simulink model "six_phase_plant"  (R2024b)
settings: Solver=FixedStepAuto  StartTime=0  StopTime=Tend  FixedStep=Tsim  RelTol=1e-3
values from neighbouring files (symbols this model uses):
  alpha_s = 2*pi/m*ps    (= 5.23598775598)    [setup.m]
  alpha_t = 2*pi/m*p    (= 4.18879020479)    [setup.m]
  Cm = 2/m    (= 0.333333333333)    [setup.m]
  fx_cmd = 9    [setup.m]
  fx_end = 0.025    [setup.m]
  fx_start = 0.002    [setup.m]
  fy_cmd = -4.5    [setup.m]
  fy_end = 0.025    [setup.m]
  fy_start = 0.001    [setup.m]
  id_cmd = 0    [setup.m]
  id_end = 0.025    [setup.m]
  id_start = 0    [setup.m]
  Ke = 0.003    [setup.m]
  Kf = 1.8    [setup.m]
  Ki_s = R*wb    (= 942.477796077)    [setup.m]
  Ki_t = R*wb    (= 942.477796077)    [setup.m]
  Kp_s = Ls*wb    (= 1.41371669412)    [setup.m]
  Kp_t = Lt*wb    (= 0.942477796077)    [setup.m]
  Kt = 0.02    [setup.m]
  Ls = L_alpha_beta(3,3)    [setup.m]
  Lt = L_alpha_beta(1,1)    [setup.m]
  p = 4    [setup.m]
  speed_cmd = 7500    [setup.m]
  torque_cmd = 0.2    [setup.m]
  torque_end = 0.025    [setup.m]
  torque_start = 0.002    [setup.m]
settings Model: Creator=chiba  LastModifiedBy=tnoguchi
settings SolverCC: AllowMultiTaskInputOutput=on
settings OptimizationCC: DefaultParameterBehavior=Inlined  ReuseModelBlockBuffer=off  EnhancedBackFolding=on  PassReuseOutputArgsAs=Individual arguments  ZeroExternalMemoryAtStartup=off  ZeroInternalMemoryAtStartup=off  OptimizeBlockOrder=speed  DifferentSizesBufferReuse=on  EfficientTunableParamExpr=on
settings DebuggingCC: ParameterTunabilityLossMsg=error
settings SFSimCC: MATLABDynamicMemAlloc=off
settings RTWCC: Description=Embedded Coder  SystemTargetFile=ert.tlc  TemplateMakefile=ert_default_tmf  GPUComputeCapability=3.5
settings CodeAppCC: ForceParamTrailComments=on  IgnoreCustomStorageClasses=off  OperatorAnnotations=on  SimulinkDataObjDesc=on  SFDataObjDesc=on  InsertBlockDesc=on
settings ERTTargetCC: TargetLangStandard=C99 (ISO)  ERTCustomFileTemplate=example_file_process.tlc  DynamicArrayContainerType=coder::array

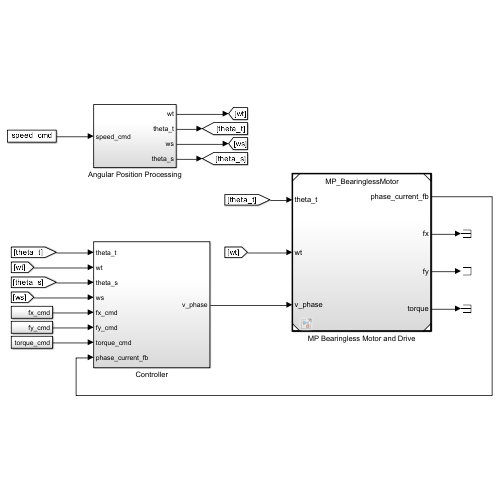
[thumbnail: Simulink's stored preview of the top-level diagram]
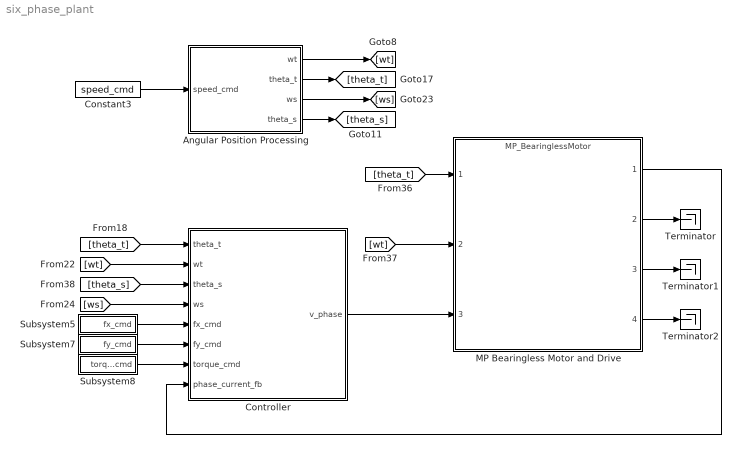
== system six_phase_plant ==
  Angular Position Processing : Subsystem
  Constant3 : Constant  Value=speed_cmd
  Controller : Subsystem
  MP Bearingless Motor and Drive : ModelReference  ModelNameDialog=MP_BearinglessMotor  SimulationMode=Normal  ModelReferenceVersion=5.215
  Subsystem5 : Subsystem
  Subsystem7 : Subsystem
  Subsystem8 : Subsystem
  Terminator : Terminator
  Terminator1 : Terminator
  Terminator2 : Terminator
  wires:
  Constant3/1 -> Angular Position Processing/1(speed_cmd)
  Angular Position Processing/1(wt) -> [wt]
  Angular Position Processing/2(theta_t) -> [theta_t]
  Angular Position Processing/3(ws) -> [ws]
  Angular Position Processing/4(theta_s) -> [theta_s]
  [wt] -> MP Bearingless Motor and Drive/2
  [theta_t] -> MP Bearingless Motor and Drive/1
  [theta_t] -> Controller/1(theta_t)
  [wt] -> Controller/2(wt)
  [theta_s] -> Controller/3(theta_s)
  [ws] -> Controller/4(ws)
  Subsystem5/1(fx_cmd) -> Controller/5(fx_cmd)
  Subsystem7/1(fy_cmd) -> Controller/6(fy_cmd)
  Subsystem8/1(torque_cmd) -> Controller/7(torque_cmd)
  Controller/1(v_phase) -> MP Bearingless Motor and Drive/3
  MP Bearingless Motor and Drive/2 -> Terminator/1
  MP Bearingless Motor and Drive/3 -> Terminator1/1
  MP Bearingless Motor and Drive/4 -> Terminator2/1
  MP Bearingless Motor and Drive/1 -> Controller/8(phase_current_fb)

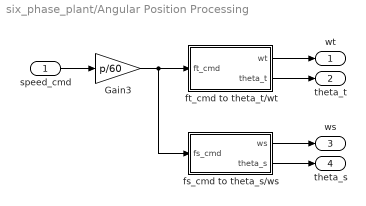
== system six_phase_plant/Angular Position Processing ==
  speed_cmd : Inport
  Gain3 : Gain  Gain=p/60
  fs_cmd to theta_s/ws : Subsystem
  ft_cmd to theta_t/wt : Subsystem
  wt : Outport
  theta_t : Outport  Port=2
  ws : Outport  Port=3
  theta_s : Outport  Port=4
  wires:
  ft_cmd to theta_t/wt/1(wt) -> wt/1
  fs_cmd to theta_s/ws/1(ws) -> ws/1
  Gain3/1 -> fs_cmd to theta_s/ws/1(fs_cmd), ft_cmd to theta_t/wt/1(ft_cmd)
  speed_cmd/1 -> Gain3/1
  ft_cmd to theta_t/wt/2(theta_t) -> theta_t/1
  fs_cmd to theta_s/ws/2(theta_s) -> theta_s/1

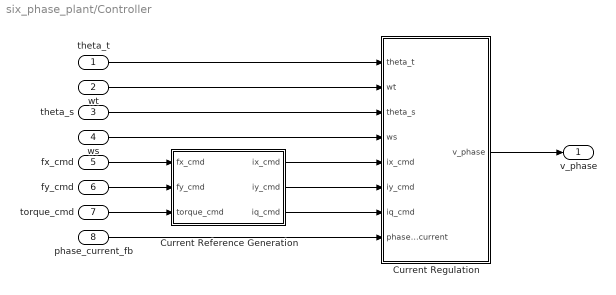
== system six_phase_plant/Controller ==
  theta_t : Inport
  wt : Inport  Port=2
  theta_s : Inport  Port=3
  ws : Inport  Port=4
  fx_cmd : Inport  Port=5
  fy_cmd : Inport  Port=6
  torque_cmd : Inport  Port=7
  phase_current_fb : Inport  Port=8
  Current Reference Generation : Subsystem
  Current Regulation : Subsystem
  v_phase : Outport
  wires:
  Current Reference Generation/3(iq_cmd) -> Current Regulation/7(iq_cmd)
  fy_cmd/1 -> Current Reference Generation/2(fy_cmd)
  torque_cmd/1 -> Current Reference Generation/3(torque_cmd)
  fx_cmd/1 -> Current Reference Generation/1(fx_cmd)
  Current Reference Generation/2(iy_cmd) -> Current Regulation/6(iy_cmd)
  theta_t/1 -> Current Regulation/1(theta_t)
  phase_current_fb/1 -> Current Regulation/8(phase_current)
  Current Regulation/1(v_phase) -> v_phase/1
  Current Reference Generation/1(ix_cmd) -> Current Regulation/5(ix_cmd)
  theta_s/1 -> Current Regulation/3(theta_s)
  ws/1 -> Current Regulation/4(ws)
  wt/1 -> Current Regulation/2(wt)

== system six_phase_plant/Subsystem5 ==
  Sum2 : Sum  Inputs=|++
  step : Step  Time=fx_start  After=fx_cmd  SampleTime=0
  step1 : Step  Time=fx_end  After=-fx_cmd  SampleTime=0
  fx_cmd : Outport
  wires:
  step1/1 -> Sum2/2
  step/1 -> Sum2/1
  Sum2/1 -> fx_cmd/1

== system six_phase_plant/Subsystem7 ==
  Sum2 : Sum  Inputs=|++
  step : Step  Time=fy_start  After=fy_cmd  SampleTime=0
  step1 : Step  Time=fy_end  After=-fy_cmd  SampleTime=0
  fy_cmd : Outport
  wires:
  step1/1 -> Sum2/2
  step/1 -> Sum2/1
  Sum2/1 -> fy_cmd/1

== system six_phase_plant/Subsystem8 ==
  Sum2 : Sum  Inputs=|++
  step : Step  Time=torque_start  After=torque_cmd  SampleTime=0
  step1 : Step  Time=torque_end  After=-torque_cmd  SampleTime=0
  torque_cmd : Outport
  wires:
  step1/1 -> Sum2/2
  step/1 -> Sum2/1
  Sum2/1 -> torque_cmd/1

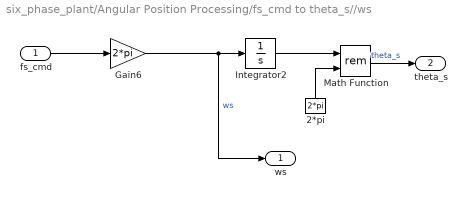
== system six_phase_plant/Angular Position Processing/fs_cmd to theta_s//ws ==
  fs_cmd : Inport
  2*pi : Constant  Value=2*pi
  Gain6 : Gain  Gain=2*pi
  Integrator2 : Integrator
  Math Function : Math  Operator=rem  SignedPower=on
  ws : Outport
  theta_s : Outport  Port=2
  wires:
  Gain6/1 -> ws/1, Integrator2/1  "ws"
  2*pi/1 -> Math Function/2
  fs_cmd/1 -> Gain6/1
  Integrator2/1 -> Math Function/1
  Math Function/1 -> theta_s/1  "theta_s"

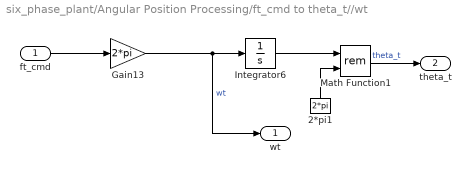
== system six_phase_plant/Angular Position Processing/ft_cmd to theta_t//wt ==
  ft_cmd : Inport
  2*pi1 : Constant  Value=2*pi
  Gain13 : Gain  Gain=2*pi
  Integrator6 : Integrator
  Math Function1 : Math  Operator=rem  SignedPower=on
  wt : Outport
  theta_t : Outport  Port=2
  wires:
  Integrator6/1 -> Math Function1/1
  ft_cmd/1 -> Gain13/1
  2*pi1/1 -> Math Function1/2
  Gain13/1 -> wt/1, Integrator6/1  "wt"
  Math Function1/1 -> theta_t/1  "theta_t"

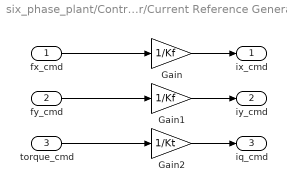
== system six_phase_plant/Controller/Current Reference Generation ==
  fx_cmd : Inport
  fy_cmd : Inport  Port=2
  torque_cmd : Inport  Port=3
  Gain : Gain  Gain=1/Kf
  Gain1 : Gain  Gain=1/Kf
  Gain2 : Gain  Gain=1/Kt
  ix_cmd : Outport
  iy_cmd : Outport  Port=2
  iq_cmd : Outport  Port=3
  wires:
  fx_cmd/1 -> Gain/1
  Gain2/1 -> iq_cmd/1
  Gain1/1 -> iy_cmd/1
  fy_cmd/1 -> Gain1/1
  torque_cmd/1 -> Gain2/1
  Gain/1 -> ix_cmd/1

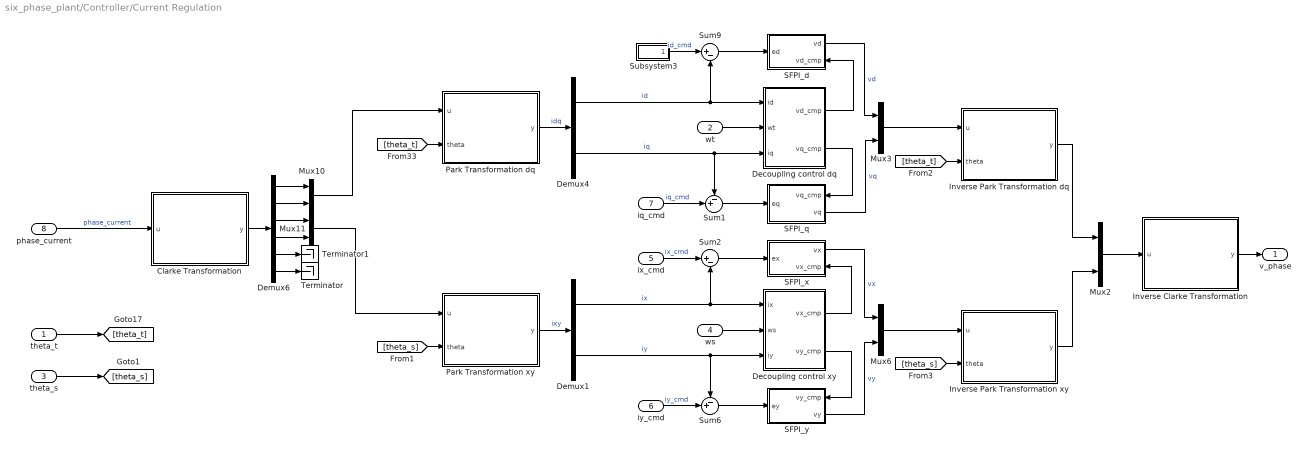
== system six_phase_plant/Controller/Current Regulation ==
  theta_t : Inport
  wt : Inport  Port=2
  theta_s : Inport  Port=3
  ws : Inport  Port=4
  ix_cmd : Inport  Port=5
  iy_cmd : Inport  Port=6
  iq_cmd : Inport  Port=7
  phase_current : Inport  Port=8
  Clarke Transformation : MATLAB Function  TreatAsAtomicUnit=on
  Decoupling control dq : Subsystem
  Decoupling control xy : Subsystem
  Demux1 : Demux  Outputs=2
  Demux4 : Demux  Outputs=2
  Demux6 : Demux  Outputs=6
  Inverse Clarke Transformation : MATLAB Function  TreatAsAtomicUnit=on
  Inverse Park Transformation dq : MATLAB Function  TreatAsAtomicUnit=on
  Inverse Park Transformation xy : MATLAB Function  TreatAsAtomicUnit=on
  Mux{2..3,6,10..11} (5 alike) : Mux  Inputs=2
  Park Transformation dq : MATLAB Function  TreatAsAtomicUnit=on
  Park Transformation xy : MATLAB Function  TreatAsAtomicUnit=on
  SFPI_d : Subsystem
      settings: PortSchema="{\"entries\":[{\"content\":{\"sides\":[{\"content\":{\"connectorIds\":[\"In1\"]},\"type\":\"ConnectorPlacement.EquallySpacedRectSide\",\"uuid\":\"0c9b1a56-be5b-4008-a4be-2c96991c93df\"},{\"content\":{\"connectorIds\":[\"Out1\",\"In2\"],\"side\":\"RIGHT\"},\"type\":\"ConnectorPlacement.EquallySpacedRectSide\",\"uuid\":\"62f10227-e6d2-436b-83cf-88635ef632ae\"},{\"content\":{\"side\":\"TOP\"},\"type\":\"ConnectorPlacement.EquallySpacedRectSide\",\"uuid\":\"775f088e-b169-44e0-8f62-950b5ccb7049\"}]},\"type\":\"ConnectorPlacement.EquallySpacedConnector\",\"uuid\":\"a91bb4f4-db64-42d6-b57d-9e899cd3ff7e\"}],\"packageUris\":[\"http://schema.mathworks.com/mf0/Connector/R2020b\"],\"version\":\"1.0\"}"
  SFPI_q : Subsystem
      settings: PortSchema="{\"entries\":[{\"content\":{\"sides\":[{\"content\":{\"connectorIds\":[\"In1\"]},\"type\":\"ConnectorPlacement.EquallySpacedRectSide\",\"uuid\":\"0c9b1a56-be5b-4008-a4be-2c96991c93df\"},{\"content\":{\"connectorIds\":[\"In2\",\"Out1\"],\"side\":\"RIGHT\"},\"type\":\"ConnectorPlacement.EquallySpacedRectSide\",\"uuid\":\"62f10227-e6d2-436b-83cf-88635ef632ae\"},{\"content\":{\"side\":\"TOP\"},\"type\":\"ConnectorPlacement.EquallySpacedRectSide\",\"uuid\":\"775f088e-b169-44e0-8f62-950b5ccb7049\"}]},\"type\":\"ConnectorPlacement.EquallySpacedConnector\",\"uuid\":\"a91bb4f4-db64-42d6-b57d-9e899cd3ff7e\"}],\"packageUris\":[\"http://schema.mathworks.com/mf0/Connector/R2020b\"],\"version\":\"1.0\"}"
  SFPI_x : Subsystem
      settings: PortSchema="{\"entries\":[{\"content\":{\"sides\":[{\"content\":{\"connectorIds\":[\"In1\"]},\"type\":\"ConnectorPlacement.EquallySpacedRectSide\",\"uuid\":\"0c9b1a56-be5b-4008-a4be-2c96991c93df\"},{\"content\":{\"connectorIds\":[\"Out1\",\"In2\"],\"side\":\"RIGHT\"},\"type\":\"ConnectorPlacement.EquallySpacedRectSide\",\"uuid\":\"62f10227-e6d2-436b-83cf-88635ef632ae\"},{\"content\":{\"side\":\"TOP\"},\"type\":\"ConnectorPlacement.EquallySpacedRectSide\",\"uuid\":\"775f088e-b169-44e0-8f62-950b5ccb7049\"}]},\"type\":\"ConnectorPlacement.EquallySpacedConnector\",\"uuid\":\"a91bb4f4-db64-42d6-b57d-9e899cd3ff7e\"}],\"packageUris\":[\"http://schema.mathworks.com/mf0/Connector/R2020b\"],\"version\":\"1.0\"}"
  SFPI_y : Subsystem
      settings: PortSchema="{\"entries\":[{\"content\":{\"sides\":[{\"content\":{\"connectorIds\":[\"In1\"]},\"type\":\"ConnectorPlacement.EquallySpacedRectSide\",\"uuid\":\"0c9b1a56-be5b-4008-a4be-2c96991c93df\"},{\"content\":{\"connectorIds\":[\"In2\",\"Out1\"],\"side\":\"RIGHT\"},\"type\":\"ConnectorPlacement.EquallySpacedRectSide\",\"uuid\":\"62f10227-e6d2-436b-83cf-88635ef632ae\"},{\"content\":{\"side\":\"TOP\"},\"type\":\"ConnectorPlacement.EquallySpacedRectSide\",\"uuid\":\"775f088e-b169-44e0-8f62-950b5ccb7049\"}]},\"type\":\"ConnectorPlacement.EquallySpacedConnector\",\"uuid\":\"a91bb4f4-db64-42d6-b57d-9e899cd3ff7e\"}],\"packageUris\":[\"http://schema.mathworks.com/mf0/Connector/R2020b\"],\"version\":\"1.0\"}"
  Subsystem3 : Subsystem
  Sum1 : Sum  Inputs=-+|
  Sum2 : Sum  Inputs=|+-
  Sum6 : Sum  Inputs=-+|
  Sum9 : Sum  Inputs=|+-
  Terminator : Terminator
  Terminator1 : Terminator
  v_phase : Outport
  wires:
  Park Transformation dq/1(y) -> Demux4/1  "idq"
  Demux6/1 -> Mux10/1
  Decoupling control dq/1(vd_cmp) -> SFPI_d/2(vd_cmp)
  ws/1 -> Decoupling control xy/2(ws)
  SFPI_y/1(vy) -> Mux6/2  "vy"
  Decoupling control dq/2(vq_cmp) -> SFPI_q/2(vq_cmp)
  Decoupling control xy/1(vx_cmp) -> SFPI_x/2(vx_cmp)
  Demux1/2 -> Sum6/1, Decoupling control xy/3(iy)  "iy"
  Mux2/1 -> Inverse Clarke Transformation/1(u)
  Mux3/1 -> Inverse Park Transformation dq/1(u)
  Mux11/1 -> Park Transformation xy/1(u)
  Mux6/1 -> Inverse Park Transformation xy/1(u)
  Demux6/3 -> Mux11/1
  Sum6/1 -> SFPI_y/1(ey)
  Demux6/4 -> Mux11/2
  Demux4/1 -> Sum9/2, Decoupling control dq/1(id)  "id"
  Decoupling control xy/2(vy_cmp) -> SFPI_y/2(vy_cmp)
  phase_current/1 -> Clarke Transformation/1(u)  "phase_current"
  Demux1/1 -> Sum2/2, Decoupling control xy/1(ix)  "ix"
  SFPI_x/1(vx) -> Mux6/1  "vx"
  SFPI_q/1(vq) -> Mux3/2  "vq"
  ix_cmd/1 -> Sum2/1  "ix_cmd"
  Demux6/5 -> Terminator1/1
  Demux4/2 -> Sum1/1, Decoupling control dq/3(iq)  "iq"
  Sum9/1 -> SFPI_d/1(ed)
  Inverse Park Transformation dq/1(y) -> Mux2/1
  iq_cmd/1 -> Sum1/2  "iq_cmd"
  Sum2/1 -> SFPI_x/1(ex)
  Demux6/6 -> Terminator/1
  Inverse Park Transformation xy/1(y) -> Mux2/2
  [theta_s] -> Park Transformation xy/2(theta)
  Subsystem3/1(id_cmd) -> Sum9/1  "id_cmd"
  Park Transformation xy/1(y) -> Demux1/1  "ixy"
  SFPI_d/1(vd) -> Mux3/1  "vd"
  Mux10/1 -> Park Transformation dq/1(u)
  Demux6/2 -> Mux10/2
  Sum1/1 -> SFPI_q/1(eq)
  Clarke Transformation/1(y) -> Demux6/1
  wt/1 -> Decoupling control dq/2(wt)
  [theta_t] -> Park Transformation dq/2(theta)
  iy_cmd/1 -> Sum6/2  "iy_cmd"
  Inverse Clarke Transformation/1(y) -> v_phase/1
  [theta_t] -> Inverse Park Transformation dq/2(theta)
  [theta_s] -> Inverse Park Transformation xy/2(theta)
  theta_t/1 -> [theta_t]
  theta_s/1 -> [theta_s]

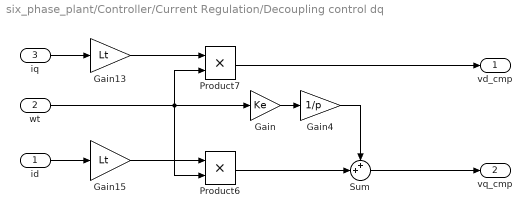
== system six_phase_plant/Controller/Current Regulation/Decoupling control dq ==
  id : Inport
  wt : Inport  Port=2
  iq : Inport  Port=3
  Gain : Gain  Gain=Ke
  Gain13 : Gain  Gain=Lt
  Gain15 : Gain  Gain=Lt
  Gain4 : Gain  Gain=1/p
  Product6 : Product
  Product7 : Product
  Sum : Sum  Inputs=++|
  vd_cmp : Outport
  vq_cmp : Outport  Port=2
  wires:
  Gain15/1 -> Product6/1
  Gain13/1 -> Product7/1
  Product7/1 -> vd_cmp/1
  id/1 -> Gain15/1
  iq/1 -> Gain13/1
  Gain/1 -> Gain4/1
  wt/1 -> Gain/1, Product7/2, Product6/2
  Product6/1 -> Sum/2
  Sum/1 -> vq_cmp/1
  Gain4/1 -> Sum/1

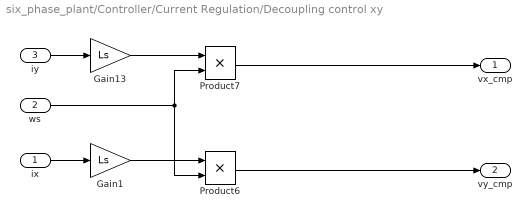
== system six_phase_plant/Controller/Current Regulation/Decoupling control xy ==
  ix : Inport
  ws : Inport  Port=2
  iy : Inport  Port=3
  Gain1 : Gain  Gain=Ls
  Gain13 : Gain  Gain=Ls
  Product6 : Product
  Product7 : Product
  vx_cmp : Outport
  vy_cmp : Outport  Port=2
  wires:
  Gain1/1 -> Product6/1
  ws/1 -> Product7/2, Product6/2
  Gain13/1 -> Product7/1
  Product7/1 -> vx_cmp/1
  ix/1 -> Gain1/1
  iy/1 -> Gain13/1
  Product6/1 -> vy_cmp/1

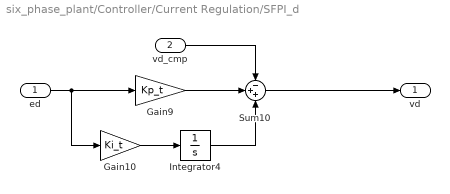
== system six_phase_plant/Controller/Current Regulation/SFPI_d ==
  ed : Inport
  vd_cmp : Inport  Port=2
  Gain10 : Gain  Gain=Ki_t
  Gain9 : Gain  Gain=Kp_t
  Integrator4 : Integrator
  Sum10 : Sum  Inputs=-++
  vd : Outport
  wires:
  vd_cmp/1 -> Sum10/1
  Gain10/1 -> Integrator4/1
  Gain9/1 -> Sum10/2
  Sum10/1 -> vd/1
  ed/1 -> Gain10/1, Gain9/1
  Integrator4/1 -> Sum10/3

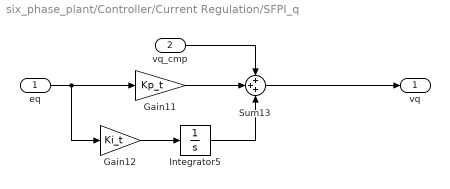
== system six_phase_plant/Controller/Current Regulation/SFPI_q ==
  eq : Inport
  vq_cmp : Inport  Port=2
  Gain11 : Gain  Gain=Kp_t
  Gain12 : Gain  Gain=Ki_t
  Integrator5 : Integrator
  Sum13 : Sum  Inputs=+++
  vq : Outport
  wires:
  eq/1 -> Gain12/1, Gain11/1
  Gain12/1 -> Integrator5/1
  Sum13/1 -> vq/1
  Integrator5/1 -> Sum13/3
  Gain11/1 -> Sum13/2
  vq_cmp/1 -> Sum13/1

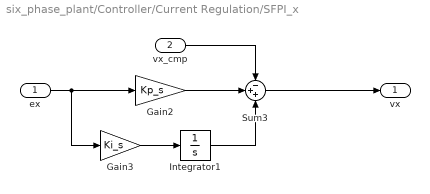
== system six_phase_plant/Controller/Current Regulation/SFPI_x ==
  ex : Inport
  vx_cmp : Inport  Port=2
  Gain2 : Gain  Gain=Kp_s
  Gain3 : Gain  Gain=Ki_s
  Integrator1 : Integrator
  Sum3 : Sum  Inputs=-++
  vx : Outport
  wires:
  Gain3/1 -> Integrator1/1
  ex/1 -> Gain3/1, Gain2/1
  Gain2/1 -> Sum3/2
  Integrator1/1 -> Sum3/3
  Sum3/1 -> vx/1
  vx_cmp/1 -> Sum3/1

== system six_phase_plant/Controller/Current Regulation/SFPI_y ==
  ey : Inport
  vy_cmp : Inport  Port=2
  Gain7 : Gain  Gain=Kp_s
  Gain8 : Gain  Gain=Ki_s
  Integrator3 : Integrator
  Sum1 : Sum  Inputs=+++
  vy : Outport
  wires:
  Integrator3/1 -> Sum1/3
  vy_cmp/1 -> Sum1/1
  Sum1/1 -> vy/1
  ey/1 -> Gain8/1, Gain7/1
  Gain8/1 -> Integrator3/1
  Gain7/1 -> Sum1/2

== system six_phase_plant/Controller/Current Regulation/Subsystem3 ==
  Sum2 : Sum  Inputs=|++
  step : Step  Time=id_start  After=id_cmd  SampleTime=0
  step1 : Step  Time=id_end  After=-id_cmd  SampleTime=0
  id_cmd : Outport
  wires:
  step1/1 -> Sum2/2
  step/1 -> Sum2/1
  Sum2/1 -> id_cmd/1

== matlab function six_phase_plant/Controller/Current Regulation/Inverse Park Transformation dq ==
  data: u input; y output; theta input
function y  = fcn(u,theta)

ab = [cos(theta) -sin(theta); sin(theta) cos(theta)]*u;

alpha = ab(1);
beta = ab(2);
y = [alpha; beta];

== matlab function six_phase_plant/Controller/Current Regulation/Inverse Park Transformation xy ==
  data: u input; y output; theta input
function y  = fcn(u,theta)

ab = [cos(theta) -sin(theta); sin(theta) cos(theta)]*u;

alpha = ab(1);
beta = ab(2);
y = [alpha; beta];

== matlab function six_phase_plant/Controller/Current Regulation/Park Transformation dq ==
  data: u input; y output; theta input
function y  = fcn(u,theta)

dq = [cos(theta) sin(theta); -sin(theta) cos(theta)]*u;

d = dq(1);
q = dq(2);
y = [d; q];

== matlab function six_phase_plant/Controller/Current Regulation/Park Transformation xy ==
  data: u input; y output; theta input
function y  = fcn(u,theta)

dq = [cos(theta) sin(theta); -sin(theta) cos(theta)]*u;

d = dq(1);
q = dq(2);
y = [d; q];

== matlab function six_phase_plant/Controller/Current Regulation/Inverse Clarke Transformation ==
  data: u input; y output; alpha_t parameter; alpha_s parameter; Cm parameter
function y = fcn(u, alpha_t, alpha_s, Cm)

u = [u; 0; 0];
Clarke = Cm*[cos(0*alpha_t) cos(1*alpha_t) cos(2*alpha_t) cos(3*alpha_t) cos(4*alpha_t) cos(5*alpha_t);
             sin(0*alpha_t) sin(1*alpha_t) sin(2*alpha_t) sin(3*alpha_t) sin(4*alpha_t) sin(5*alpha_t);
             cos(0*alpha_s) cos(1*alpha_s) cos(2*alpha_s) cos(3*alpha_s) cos(4*alpha_s) cos(5*alpha_s);
             sin(0*alpha_s) sin(1*alpha_s) sin(2*alpha_s) sin(3*alpha_s) sin(4*alpha_s) sin(5*alpha_s);
             1 1 1 1 1 1;
             1 -1 1 -1 1 -1;];

y = Clarke\u;  % equivalent to inv(Clarke)*u

end

== matlab function six_phase_plant/Controller/Current Regulation/Clarke Transformation ==
  data: u input; y output; alpha_t parameter; alpha_s parameter; Cm parameter
function y = fcn(u, alpha_t, alpha_s, Cm)

Clarke = Cm*[cos(0*alpha_t) cos(1*alpha_t) cos(2*alpha_t) cos(3*alpha_t) cos(4*alpha_t) cos(5*alpha_t);
             sin(0*alpha_t) sin(1*alpha_t) sin(2*alpha_t) sin(3*alpha_t) sin(4*alpha_t) sin(5*alpha_t);
             cos(0*alpha_s) cos(1*alpha_s) cos(2*alpha_s) cos(3*alpha_s) cos(4*alpha_s) cos(5*alpha_s);
             sin(0*alpha_s) sin(1*alpha_s) sin(2*alpha_s) sin(3*alpha_s) sin(4*alpha_s) sin(5*alpha_s);
             1 1 1 1 1 1;
             1 -1 1 -1 1 -1;];

y = Clarke*u;

end
